simulink model "qpsk_ascii_system"  (R2022b)
settings: Solver=FixedStepDiscrete  StartTime=0.0  StopTime=0  RelTol=1e-3
model workspace (MAT data in the model file):
  simulinkFilterSpan = 10
  simulinkNoiseSeed = 1201
  simulinkRolloff = 0.35
  simulinkSNRdB = 23.9794000867
  simulinkSampleIndices = [81 89 97 105 113 121 129 137 145 153 161 169 177 185 193 201 209 217 225 233 241 249 257 265 273 281 289 297 305 313 321 329 337 345 353 361]
  simulinkSps = 8
  simulinkWaveformLength = 368
  txBitsIn = [0; 1; 0; 0; 1; 0; 0; 0; 0; 1; 0; 0; 0; 1; 0; 1; 0; 1; 0; 0; 1; 1; 0; 0; 0; 1; 0; 0; 1; 1; 0; 0; 0; 1; 0; 0; 1; 1; 1; 1; 0; 0; 1; 0; 0; 0; 0; 0; 0; 1; 0; 0; 1; 0; 0; 0; 0; 1; 0; 0; 0; 1; 0; 1; 0; 1; 0; 1; 0; 1; 0; 1; 0; 0; 0; 0; 0; 0; 0; 0; 0; 0; 0; 0; 0; 0; 0; 0; 0; 0; 0; 0]
libraries: commdigbbndpm3 x2, commfilt2 x2, commchan3 x1
Description:
  | QPSK ASCII communication chain for MATLAB R2022b.
  | ASCII conversion and final text verification are performed by run_simulink_demo.m; all physical-link stages run in this model.
settings Model: Creator=Dell  LastModifiedBy=Dell
settings DataIOCC: SaveOutput=off  SignalLogging=off

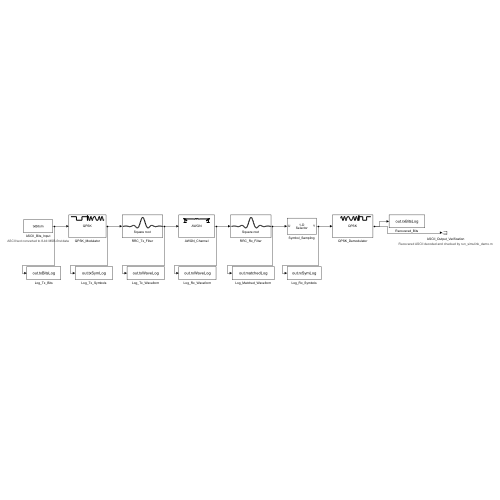
[thumbnail: Simulink's stored preview of the top-level diagram]
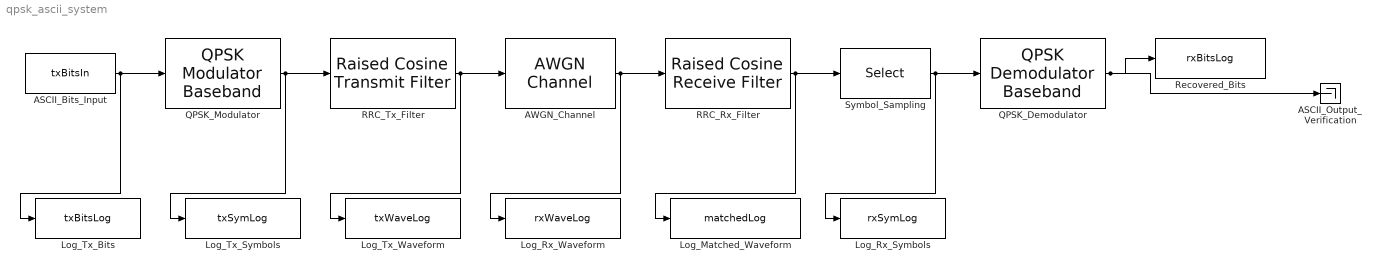
== system qpsk_ascii_system ==
  ASCII_Bits_Input : Constant  Value=txBitsIn
      settings: AttributesFormatString=ASCII text converted to 8-bit MSB-first data
  ASCII_Output_Verification : Terminator
      settings: AttributesFormatString=Recovered ASCII decoded and checked by run_simulink_demo.m
  AWGN_Channel : commchan3/AWGN Channel  InputProcessing=Columns as channels (frame based)  seed=simulinkNoiseSeed  noiseMode="Signal to noise ratio  (SNR)"  EbNodB=10  EsNodB=10  SNRdB=simulinkSNRdB  bitsPerSym=1  Ps=1  Tsym=1  variance=1
  Log_Matched_Waveform : ToWorkspace  VariableName=matchedLog  SampleTime=-1
  Log_Rx_Symbols : ToWorkspace  VariableName=rxSymLog  SampleTime=-1
  Log_Rx_Waveform : ToWorkspace  VariableName=rxWaveLog  SampleTime=-1
  Log_Tx_Bits : ToWorkspace  VariableName=txBitsLog  SampleTime=-1
  Log_Tx_Symbols : ToWorkspace  VariableName=txSymLog  SampleTime=-1
  Log_Tx_Waveform : ToWorkspace  VariableName=txWaveLog  SampleTime=-1
  QPSK_Demodulator : commdigbbndpm3/QPSK Demodulator Baseband  OutType=Bit  DecType=Hard decision  VarSource=Dialog  Variance=1  Dec=Gray  Ph=pi/4  outDtype1=Inherit via internal rule  outDtype2=Inherit via internal rule  derotateFactorWordLen=16  derotateFactorDataTypeStr=Inherit: Same word length as input  derotateFactorLastDataTypeStr=Inherit: Same word length as input
  QPSK_Modulator : commdigbbndpm3/QPSK Modulator Baseband  InType=Bit  Enc=Gray  Ph=pi/4  outDtype=double  outWordLen=16  outUDDataType=sfix(16)  outFracLenMode=Best precision  outFracLen=15  outDataTypeStr=double  outLastDataTypeStr=double
  RRC_Rx_Filter : commfilt2/Raised Cosine Receive Filter  filtType=Square root  R=simulinkRolloff  filtSpan=simulinkFilterSpan  N=simulinkSps  downFactor=1  downOffset=0  filterGain=1  InputProcessing=Columns as channels (frame based)  RateOptions=Enforce single-rate processing  framing=Mute  checkCoeff=off  variableName=rcRxFilt  currentFiltSpan=10  D=5  inputOffset=0  sampMode=Mute  saveAsFlag=0  rateMode=Downsampling  checkGain=Normalized  launchFVT=on  roundingMode=Floor  overflowMode=off  coeffDataTypeStr=Inherit: Same word length as input  coeffMin=[]  coeffMax=[]  coeffLastDataTypeStr=Inherit: Same word length as input  accumDataTypeStr=Inherit: Same as product output  accumLastDataTypeStr=Inherit: Same as product output  outputDataTypeStr=Inherit: Same as accumulator  outputMin=[]  outputMax=[]  outputLastDataTypeStr=Inherit: Same as accumulator
  RRC_Tx_Filter : commfilt2/Raised Cosine Transmit Filter  filtType=Square root  R=simulinkRolloff  filtSpan=simulinkFilterSpan  N=simulinkSps  filterGain=1  InputProcessing=Columns as channels (frame based)  RateOptions=Enforce single-rate processing  framing=Mute  checkCoeff=off  variableName=rcTxFilt  checkGain=Normalized  sampMode=Mute  saveAsFlag=0  currentFiltSpan=10  D=(10)/2  launchFVT=on  roundingMode=Floor  overflowMode=off  coeffDataTypeStr=Inherit: Same word length as input  coeffMin=[]  coeffMax=[]  coeffLastDataTypeStr=Inherit: Same word length as input  outputDataTypeStr=Inherit: Same as accumulator  outputMin=[]  outputMax=[]  outputLastDataTypeStr=Inherit: Same as accumulator
  Recovered_Bits : ToWorkspace  VariableName=rxBitsLog  SampleTime=-1
  Symbol_Sampling : Selector  InputPortWidth=simulinkWaveformLength  IndexOptions=Index vector (dialog)  Indices=simulinkSampleIndices  OutputSizes=numel(simulinkSampleIndices)
  wires:
  ASCII_Bits_Input/1 -> QPSK_Modulator/1, Log_Tx_Bits/1
  QPSK_Modulator/1 -> RRC_Tx_Filter/1, Log_Tx_Symbols/1
  RRC_Tx_Filter/1 -> AWGN_Channel/1, Log_Tx_Waveform/1
  AWGN_Channel/1 -> RRC_Rx_Filter/1, Log_Rx_Waveform/1
  RRC_Rx_Filter/1 -> Symbol_Sampling/1, Log_Matched_Waveform/1
  Symbol_Sampling/1 -> QPSK_Demodulator/1, Log_Rx_Symbols/1
  QPSK_Demodulator/1 -> Recovered_Bits/1, ASCII_Output_Verification/1
